simulink model "PROJEKT"  (R2023b)
settings: Solver=ode23t  StartTime=0.0  StopTime=sim_time  MaxStep=2.0  RelTol=1e-3
model workspace (MAT data in the model file):
  Upv = 0.5
undefined symbols (not defined in the file or in its folder): Ci, Cu, D1, D2, L, pv_data, pv_eq, RL, Rt, Sample, sim_time, T, U_pv_oc, Uoc_max
settings Model: Creator=teo  LastModifiedBy=teo

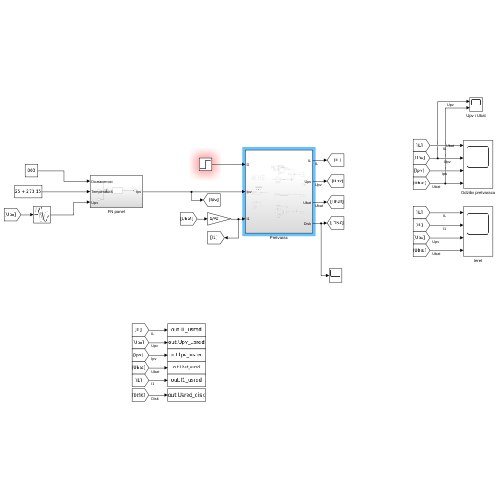
[thumbnail: Simulink's stored preview of the top-level diagram]
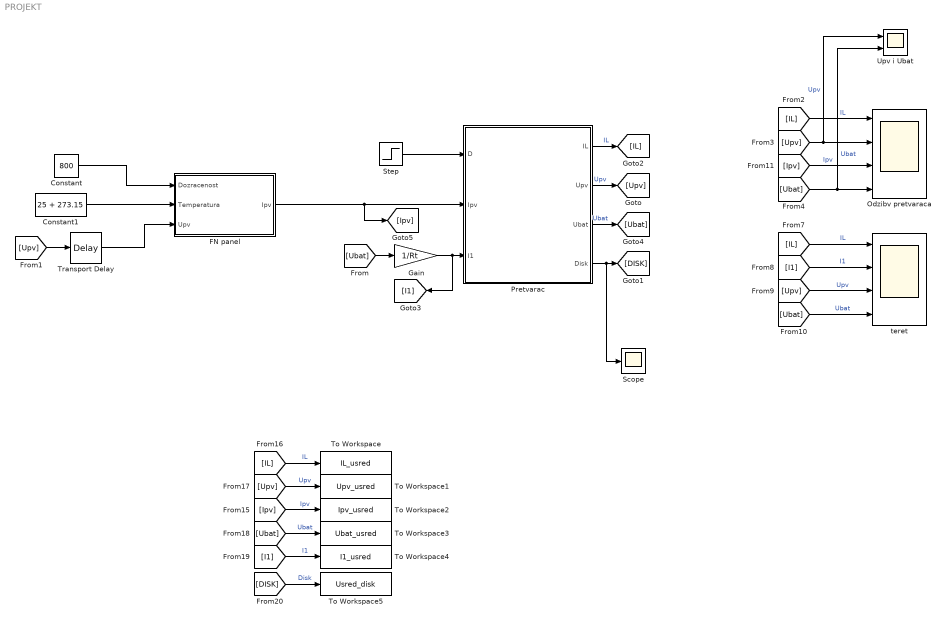
== system PROJEKT ==
  Constant : Constant  Value=800
  Constant1 : Constant  Value=25 + 273.15
  FN panel : Subsystem
  Gain : Gain  Gain=1/Rt
  Odzibv pretvaraca : Scope  NumInputPorts=4
  Pretvarac : Subsystem
  Scope : Scope
  Step : Step  Time=sim_time/2  Before=D1  After=D2  SampleTime=0
  To Workspace : ToWorkspace  VariableName=IL_usred  SaveFormat=Timeseries  SampleTime=-1
  To Workspace1 : ToWorkspace  VariableName=Upv_usred  SaveFormat=Timeseries  SampleTime=-1
  To Workspace2 : ToWorkspace  VariableName=Ipv_usred  SaveFormat=Timeseries  SampleTime=-1
  To Workspace3 : ToWorkspace  VariableName=Ubat_usred  SaveFormat=Timeseries  SampleTime=-1
  To Workspace4 : ToWorkspace  VariableName=I1_usred  SaveFormat=Timeseries  SampleTime=-1
  To Workspace5 : ToWorkspace  VariableName=Usred_disk  SaveFormat=Timeseries  SampleTime=-1
  Transport Delay : TransportDelay  DelayTime=0.0001
  Upv i Ubat : Scope  NumInputPorts=2
  teret : Scope  NumInputPorts=4
  wires:
  Pretvarac/1(IL) -> [IL]  "IL"
  Pretvarac/2(Upv) -> [Upv]  "Upv"
  Pretvarac/3(Ubat) -> [Ubat]  "Ubat"
  Pretvarac/4(Disk) -> Scope/1, [DISK]
  FN panel/1(Ipv) -> [Ipv], Pretvarac/2(Ipv)
  Gain/1 -> [I1], Pretvarac/3(I1)
  [Ubat] -> Gain/1
  Transport Delay/1 -> FN panel/3(Upv)
  Constant/1 -> FN panel/1(Dozracenost)
  Constant1/1 -> FN panel/2(Temperatura)
  [Upv] -> Transport Delay/1
  Step/1 -> Pretvarac/1(D)
  [Ubat] -> Upv i Ubat/2, Odzibv pretvaraca/4  "Ubat"
  [IL] -> Odzibv pretvaraca/1  "IL"
  [Upv] -> Upv i Ubat/1, Odzibv pretvaraca/2  "Upv"
  [I1] -> teret/2  "I1"
  [Ubat] -> teret/4  "Ubat"
  [Ipv] -> Odzibv pretvaraca/3  "Ipv"
  [IL] -> teret/1  "IL"
  [Upv] -> teret/3  "Upv"
  [Ubat] -> To Workspace3/1  "Ubat"
  [Ipv] -> To Workspace2/1  "Ipv"
  [Upv] -> To Workspace1/1  "Upv"
  [I1] -> To Workspace4/1  "I1"
  [IL] -> To Workspace/1  "IL"
  [DISK] -> To Workspace5/1  "Disk"

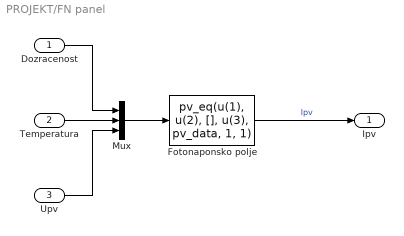
== system PROJEKT/FN panel ==
  Dozracenost : Inport
  Temperatura : Inport  Port=2
  Upv : Inport  Port=3
  Fotonaponsko polje : MATLABFcn  MATLABFcn=pv_eq(u(1), u(2), [], u(3), pv_data, 1, 1)  OutputDimensions=1
  Mux : Mux  Inputs=3
  Ipv : Outport
  wires:
  Fotonaponsko polje/1 -> Ipv/1  "Ipv"
  Mux/1 -> Fotonaponsko polje/1
  Dozracenost/1 -> Mux/1
  Temperatura/1 -> Mux/2
  Upv/1 -> Mux/3

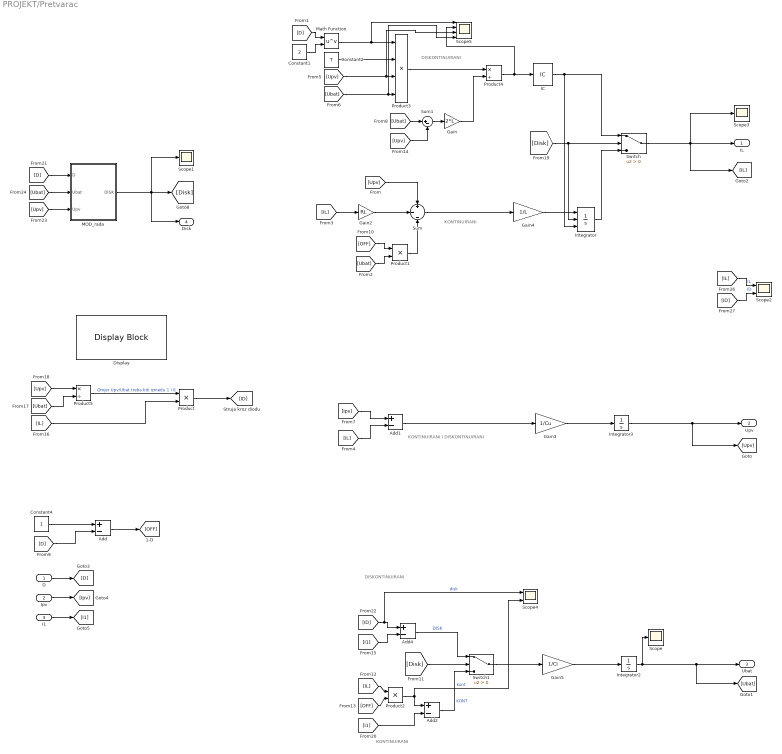
== system PROJEKT/Pretvarac ==
  note: DISKONTINUIRANI
  note: KONTINUIRANI
  note: KONTINUIRANI I DISKONTINUIRANI
  note: KONTINUIRANI
  note: DISKONTINUIRANI
  D : Inport
  Ipv : Inport  Port=2
  I1 : Inport  Port=3
  Add{,1..2,4} (4 alike) : Sum  Inputs=+-
  Constant1 : Constant  Value=2
  Constant2 : Constant  Value=T
  Constant4 : Constant
  Display : DisplayBlock  LabelPosition=Bottom  Transparency=1
  Gain : Gain  Gain=2*L
  Gain2 : Gain  Gain=RL
  Gain3 : Gain  Gain=1/Cu
  Gain4 : Gain  Gain=1/L
  Gain5 : Gain  Gain=1/Ci
  IC : InitialCondition  Value=0.1
  Integrator : Integrator  ExternalReset=falling  InitialConditionSource=external  LimitOutput=on  UpperSaturationLimit=150  LowerSaturationLimit=0
  Integrator2 : Integrator  InitialCondition=0.2  UpperSaturationLimit=Uoc_max + 10  LowerSaturationLimit=0
  Integrator3 : Integrator  InitialCondition=0.1  LimitOutput=on  UpperSaturationLimit=U_pv_oc  LowerSaturationLimit=0
  MOD_rada : Subsystem
  Math Function : Math  Operator=pow
  Product : Product
  Product1 : Product
  Product2 : Product
  Product3 : Product  Inputs=4
  Product4 : Product  Inputs=*/
  Product5 : Product  Inputs=*/
  Scope : Scope
  Scope1 : Scope
  Scope2 : Scope  NumInputPorts=2
  Scope3 : Scope
  Scope4 : Scope  NumInputPorts=2
  Scope5 : Scope  NumInputPorts=4
  Sum : Sum  Inputs=+|-|-
  Sum1 : Sum  Inputs=|+-
  Switch : Switch  Criteria=u2 > Threshold  SaturateOnIntegerOverflow=off  InputSameDT=off
  Switch1 : Switch  Criteria=u2 > Threshold  SaturateOnIntegerOverflow=off  InputSameDT=off
  IL : Outport
  Upv : Outport  Port=2
  Ubat : Outport  Port=3
  Disk : Outport  Port=4
  wires:
  I1/1 -> [I1]
  [Ipv] -> Add1/1
  D/1 -> [D]
  Ipv/1 -> [Ipv]
  [Upv] -> Sum/1
  [D] -> Add/2
  Constant4/1 -> Add/1
  Product1/1 -> Sum/3
  [OFF] -> Product1/1
  [Ubat] -> Product1/2
  [IL] -> Add1/2
  Sum/1 -> Gain4/1
  Add1/1 -> Gain3/1
  [D] -> Math Function/1
  Constant1/1 -> Math Function/2
  Math Function/1 -> Scope5/1, Product3/1
  Constant2/1 -> Product3/2
  [Upv] -> Scope5/3, Product3/3
  [Ubat] -> Scope5/4, Product3/4
  Product3/1 -> Product4/1
  [Ubat] -> Sum1/1
  [Upv] -> Sum1/2
  Sum1/1 -> Gain/1
  Gain3/1 -> Integrator3/1
  Gain/1 -> Product4/2
  Switch/1 -> Scope3/1, IL/1, [IL]
  Add/1 -> [OFF]
  Gain2/1 -> Sum/2
  [IL] -> Gain2/1
  Gain5/1 -> Integrator2/1
  [D] -> MOD_rada/1(D)
  [Upv] -> MOD_rada/3(Upv)
  [Ubat] -> MOD_rada/2(Ubat)
  Integrator3/1 -> [Upv], Upv/1
  Gain4/1 -> Integrator/1
  Integrator/1 -> Switch/3
  [Disk] -> Integrator/2, Switch/2
  [Upv] -> Product5/1
  [Ubat] -> Product5/2
  [IL] -> Product/2
  Product/1 -> [ID]
  Product5/1 -> Product/1  "Omjer Upv/Ubat treba biti izmedu 1 i 0"
  [ID] -> Scope4/1, Add4/1  "disk"
  [I1] -> Add4/2
  [IL] -> Scope2/1  "IL"
  [ID] -> Scope2/2  "ID"
  IC/1 -> Integrator/3, Switch/1
  Switch1/1 -> Gain5/1
  Add4/1 -> Switch1/1  "DISK"
  [Disk] -> Switch1/2
  [IL] -> Product2/1
  [OFF] -> Product2/2
  Product2/1 -> Add2/1, Scope4/2  "kont"
  [I1] -> Add2/2
  Add2/1 -> Switch1/3  "KONT"
  MOD_rada/1(DISK) -> Disk/1, Scope1/1, [Disk]
  Integrator2/1 -> [Ubat], Ubat/1, Scope/1
  Product4/1 -> Scope5/2, IC/1

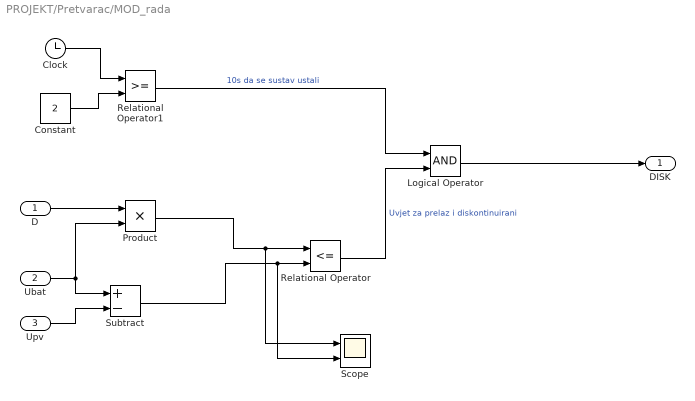
== system PROJEKT/Pretvarac/MOD_rada ==
  D : Inport  SampleTime=Sample
  Ubat : Inport  Port=2  SampleTime=Sample
  Upv : Inport  Port=3  SampleTime=Sample
  Clock : Clock
  Constant : Constant  Value=2
  Logical Operator : Logic  AllPortsSameDT=off  OutDataTypeStr=boolean
  Product : Product
  Relational Operator : RelationalOperator  Operator=<=  OutDataTypeStr=boolean  RndMeth=Simplest  InputSameDT=off
  Relational Operator1 : RelationalOperator  OutDataTypeStr=boolean  RndMeth=Simplest  InputSameDT=off
  Scope : Scope  NumInputPorts=2
  Subtract : Sum  Inputs=+-
  DISK : Outport  SampleTime=Sample
  wires:
  Ubat/1 -> Product/2, Subtract/1
  Upv/1 -> Subtract/2
  Relational Operator1/1 -> Logical Operator/1  "10s da se sustav ustali"
  Relational Operator/1 -> Logical Operator/2  "Uvjet za prelaz i diskontinuirani"
  Subtract/1 -> Scope/2, Relational Operator/2
  Product/1 -> Scope/1, Relational Operator/1
  Logical Operator/1 -> DISK/1
  Clock/1 -> Relational Operator1/1
  Constant/1 -> Relational Operator1/2
  D/1 -> Product/1
